simulink model "bdc_ang_control"  (R2018a)
settings: Solver=VariableStepAuto  StartTime=0.0  StopTime=10.0  RelTol=1e-3
model workspace (MAT data in the model file):
  Bm = 3.1346e-05
  Jm = 6.88627e-06
  Kb = 0.0583
  Ki = 0.0583
  La = 0.003694
  Ra = 5.385
settings Model: Creator=Kim  LastModifiedBy=Kim

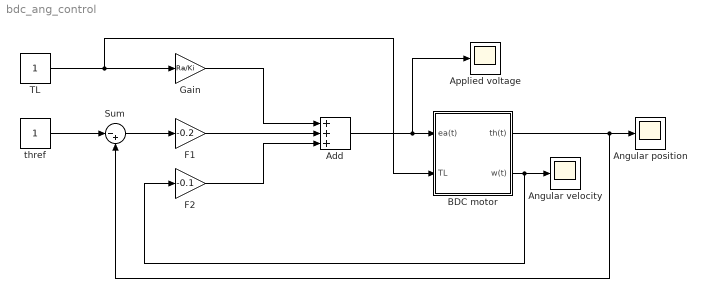
== system bdc_ang_control ==
  Add : Sum  Inputs=+++
  Angular position : Scope
  Angular velocity : Scope
  Applied voltage : Scope
  BDC motor : Subsystem
  F1 : Gain  Gain=-0.2
  F2 : Gain  Gain=-0.1
  Gain : Gain  Gain=Ra/Ki
  Sum : Sum  Inputs=|-+
  TL : Constant
  thref : Constant
  wires:
  thref/1 -> Sum/1
  BDC motor/1(th(t)) -> Angular position/1, Sum/2
  Sum/1 -> F1/1
  BDC motor/2(w(t)) -> Angular velocity/1, F2/1
  TL/1 -> BDC motor/2(TL), Gain/1
  F1/1 -> Add/2
  Gain/1 -> Add/1
  F2/1 -> Add/3
  Add/1 -> Applied voltage/1, BDC motor/1(ea(t))

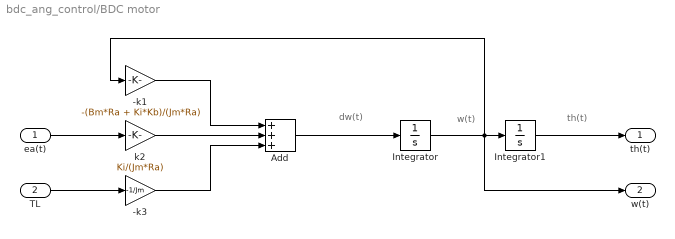
== system bdc_ang_control/BDC motor ==
  note: dw(t)
  note: w(t)
  note: th(t)
  ea(t) : Inport
  TL : Inport  Port=2
  -k1 : Gain  Gain=-(Bm*Ra + Ki*Kb)/(Jm*Ra)
  -k3 : Gain  Gain=-1/Jm
  Add : Sum  Inputs=+++
  Integrator : Integrator
  Integrator1 : Integrator
  k2 : Gain  Gain=Ki/(Jm*Ra)
  th(t) : Outport
  w(t) : Outport  Port=2
  wires:
  Integrator1/1 -> th(t)/1
  ea(t)/1 -> k2/1
  Integrator/1 -> w(t)/1, -k1/1, Integrator1/1
  -k1/1 -> Add/1
  -k3/1 -> Add/3
  TL/1 -> -k3/1
  Add/1 -> Integrator/1
  k2/1 -> Add/2
